simulink model "main_sim"  (R2021a)
settings: Solver=FixedStepAuto  StartTime=0  StopTime=11.0  FixedStep=1e-2  RelTol=1e-3
values from neighbouring files (symbols this model uses):
  Af = 1.6 + 0.00056 * (M-765)    (= 1.7316)    [main.m]    (also in perc_neg_forces.m)
  Cd = 0.27    [main.m]    (also in perc_neg_forces.m)
  Cf = Csigma    (= 40000)    [main.m]    (also in perc_neg_forces.m)
  Cr = Csigma    (= 40000)    [main.m]    (also in perc_neg_forces.m)
  f = 0.015    [main.m]    (also in perc_neg_forces.m)
  g = 9.81    [main.m]    (also in perc_neg_forces.m)
  h = 0.292*2    (= 0.584)    [main.m]    (also in perc_neg_forces.m)
  haero = 0.292*2    (= 0.584)    [main.m]    (also in perc_neg_forces.m)
  Lf = 0.74    [main.m]    (also in perc_neg_forces.m)
  Lr = 0.6    [main.m]    (also in perc_neg_forces.m)
  M = 1000    [main.m]    (also in perc_neg_forces.m)
  reff = ( asin(acos(rstat/rw)) / acos(rstat/rw)) * rw    [main.m]    (also in perc_neg_forces.m)
  rho = 1.225    [main.m]    (also in perc_neg_forces.m)
  Vwind = 5.5    [main.m]    (also in perc_neg_forces.m)
  w_cte = 5    [main.m]    (also in perc_neg_forces.m = w(i))
libraries: simulink x6
settings Model: Creator=joaofonseca  LastModifiedBy=joaofonseca

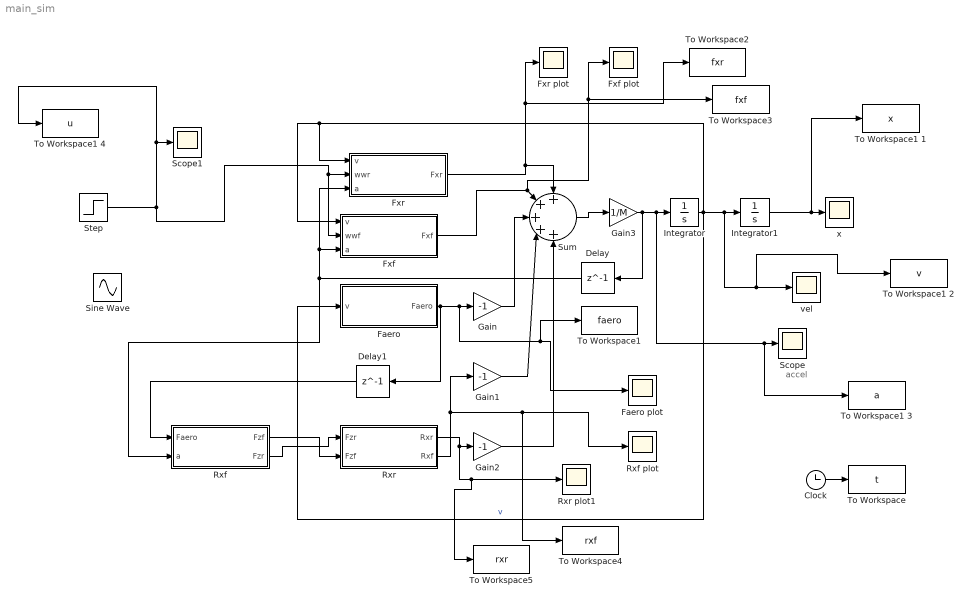
== system main_sim ==
  note: accel
  Clock : Clock
  Delay : Delay  DelayLength=1  InitialCondition=0
  Delay1 : Delay  DelayLength=1  InitialCondition=0
  Faero : Subsystem
  Faero plot : Scope
  Fxf : Subsystem
  Fxf plot : Scope
  Fxr : Subsystem
  Fxr plot : Scope
  Gain : Gain  Gain=-1
  Gain1 : Gain  Gain=-1
  Gain2 : Gain  Gain=-1
  Gain3 : Gain  Gain=1/M
  Integrator : Integrator
  Integrator1 : Integrator  InitialCondition=-2
  Rxf : Subsystem
  Rxf plot : Scope
  Rxr : Subsystem
  Rxr plot1 : Scope
  Scope : Scope
  Scope1 : Scope
  Sine Wave : Sin  Amplitude=25  Bias=26  Frequency=0.5  SampleTime=0
  Step : Step  Time=0  After=w_cte  SampleTime=0
  Sum : Sum  Inputs=+|+|+|+|+
  To Workspace : ToWorkspace  VariableName=t  SampleTime=-1
  To Workspace1 : ToWorkspace  VariableName=faero  SampleTime=-1
  To Workspace1 1 : ToWorkspace  VariableName=x  SampleTime=-1
  To Workspace1 2 : ToWorkspace  VariableName=v  SampleTime=-1
  To Workspace1 3 : ToWorkspace  VariableName=a  SampleTime=-1
  To Workspace1 4 : ToWorkspace  VariableName=u  SampleTime=-1
  To Workspace2 : ToWorkspace  VariableName=fxr  SampleTime=-1
  To Workspace3 : ToWorkspace  VariableName=fxf  SampleTime=-1
  To Workspace4 : ToWorkspace  VariableName=rxf  SampleTime=-1
  To Workspace5 : ToWorkspace  VariableName=rxr  SampleTime=-1
  vel : Scope
  x : Scope
  wires:
  Integrator/1 -> Faero/1(v), To Workspace1 2/1, vel/1, Integrator1/1, Fxf/1(v), Fxr/1(v)  "v"
  Faero/1(Faero) -> Delay1/1, To Workspace1/1, Faero plot/1, Gain/1
  Gain2/1 -> Sum/5
  Gain1/1 -> Sum/4
  Gain/1 -> Sum/3
  Fxf/1(Fxf) -> To Workspace3/1, Fxf plot/1, Sum/2
  Fxr/1(Fxr) -> To Workspace2/1, Fxr plot/1, Sum/1
  Gain3/1 -> Delay/1, To Workspace1 3/1, Scope/1, Integrator/1
  Sum/1 -> Gain3/1
  Rxr/1(Rxr) -> To Workspace5/1, Rxr plot1/1, Gain2/1
  Integrator1/1 -> To Workspace1 1/1, x/1
  Delay/1 -> Rxf/2(a), Fxf/3(a), Fxr/3(a)
  Step/1 -> Fxf/2(wwf), Fxr/2(wwr), To Workspace1 4/1, Scope1/1
  Rxf/1(Fzf) -> Rxr/2(Fzf)
  Rxf/2(Fzr) -> Rxr/1(Fzr)
  Delay1/1 -> Rxf/1(Faero)
  Rxr/2(Rxf) -> To Workspace4/1, Rxf plot/1, Gain1/1
  Clock/1 -> To Workspace/1

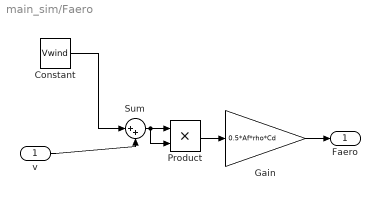
== system main_sim/Faero ==
  v : Inport
  Constant : Constant  Value=Vwind
  Gain : Gain  Gain=0.5*Af*rho*Cd
  Product : Product
  Sum : Sum  Inputs=|++
  Faero : Outport
  wires:
  Constant/1 -> Sum/1
  v/1 -> Sum/2
  Sum/1 -> Product/2, Product/1
  Product/1 -> Gain/1
  Gain/1 -> Faero/1

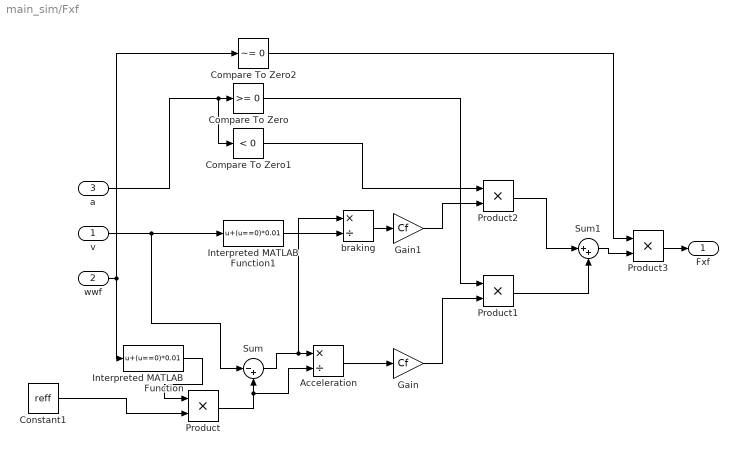
== system main_sim/Fxf ==
  v : Inport
  wwf : Inport  Port=2
  a : Inport  Port=3
  Acceleration : Product  Inputs=*/  OutMax=0.1
  Compare To Zero : simulink/Logic and Bit Operations/Compare To Zero  relop=>=  OutDataTypeStr=uint8  ZeroCross=off
  Compare To Zero1 : simulink/Logic and Bit Operations/Compare To Zero  relop=<  OutDataTypeStr=uint8  ZeroCross=off
  Compare To Zero2 : simulink/Logic and Bit Operations/Compare To Zero  relop=~=  OutDataTypeStr=uint8  ZeroCross=off
  Constant1 : Constant  Value=reff
  Gain : Gain  Gain=Cf
  Gain1 : Gain  Gain=Cf
  Interpreted MATLAB Function : MATLABFcn  MATLABFcn=u+(u==0)*0.01
  Interpreted MATLAB Function1 : MATLABFcn  MATLABFcn=u+(u==0)*0.01
  Product : Product  OutMin=0.0001
  Product1 : Product
  Product2 : Product
  Product3 : Product
  Sum : Sum  Inputs=|-+
  Sum1 : Sum  Inputs=|++
  braking : Product  Inputs=*/
  Fxf : Outport
  wires:
  Product1/1 -> Sum1/2
  Compare To Zero1/1 -> Product2/1
  Constant1/1 -> Product/2
  Product2/1 -> Sum1/1
  Product/1 -> Acceleration/2, Sum/2
  a/1 -> Compare To Zero1/1, Compare To Zero/1
  Sum/1 -> braking/1, Acceleration/1
  Compare To Zero/1 -> Product1/1
  Acceleration/1 -> Gain/1
  Gain1/1 -> Product2/2
  braking/1 -> Gain1/1
  v/1 -> Interpreted MATLAB Function1/1, Sum/1
  Gain/1 -> Product1/2
  Interpreted MATLAB Function/1 -> Product/1
  Interpreted MATLAB Function1/1 -> braking/2
  Compare To Zero2/1 -> Product3/1
  wwf/1 -> Compare To Zero2/1, Interpreted MATLAB Function/1
  Sum1/1 -> Product3/2
  Product3/1 -> Fxf/1

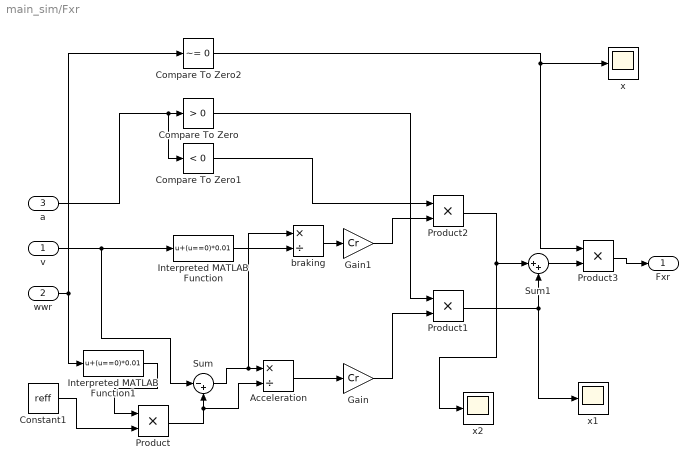
== system main_sim/Fxr ==
  v : Inport
  wwr : Inport  Port=2
  a : Inport  Port=3
  Acceleration : Product  Inputs=*/
  Compare To Zero : simulink/Logic and Bit Operations/Compare To Zero  relop=>  OutDataTypeStr=uint8  ZeroCross=off
  Compare To Zero1 : simulink/Logic and Bit Operations/Compare To Zero  relop=<  OutDataTypeStr=uint8  ZeroCross=off
  Compare To Zero2 : simulink/Logic and Bit Operations/Compare To Zero  relop=~=  OutDataTypeStr=uint8  ZeroCross=off
  Constant1 : Constant  Value=reff
  Gain : Gain  Gain=Cr
  Gain1 : Gain  Gain=Cr
  Interpreted MATLAB Function : MATLABFcn  MATLABFcn=u+(u==0)*0.01
  Interpreted MATLAB Function1 : MATLABFcn  MATLABFcn=u+(u==0)*0.01
  Product{,1..3} (4 alike) : Product
  Sum : Sum  Inputs=|-+
  Sum1 : Sum  Inputs=|++
  braking : Product  Inputs=*/
  x : Scope
  x1 : Scope
  x2 : Scope
  Fxr : Outport
  wires:
  a/1 -> Compare To Zero1/1, Compare To Zero/1
  Constant1/1 -> Product/2
  Product/1 -> Acceleration/2, Sum/2
  v/1 -> Interpreted MATLAB Function/1, Sum/1
  Sum/1 -> braking/1, Acceleration/1
  Acceleration/1 -> Gain/1
  Gain/1 -> Product1/2
  Compare To Zero/1 -> Product1/1
  Product1/1 -> x1/1, Sum1/2
  braking/1 -> Gain1/1
  Compare To Zero1/1 -> Product2/1
  Gain1/1 -> Product2/2
  Product2/1 -> x2/1, Sum1/1
  Interpreted MATLAB Function/1 -> braking/2
  wwr/1 -> Compare To Zero2/1, Interpreted MATLAB Function1/1
  Interpreted MATLAB Function1/1 -> Product/1
  Sum1/1 -> Product3/2
  Compare To Zero2/1 -> Product3/1, x/1
  Product3/1 -> Fxr/1

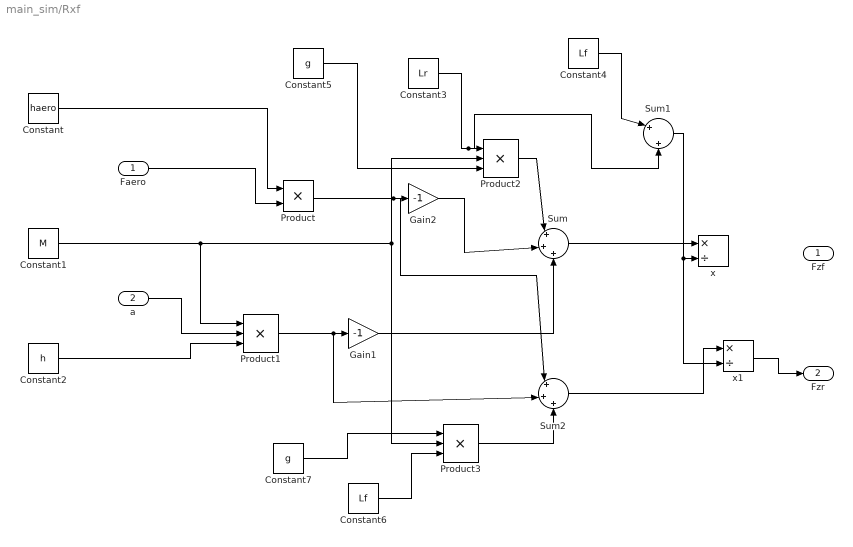
== system main_sim/Rxf ==
  Faero : Inport
  a : Inport  Port=2
  Constant : Constant  Value=haero
  Constant1 : Constant  Value=M
  Constant2 : Constant  Value=h
  Constant3 : Constant  Value=Lr
  Constant4 : Constant  Value=Lf
  Constant5 : Constant  Value=g
  Constant6 : Constant  Value=Lf
  Constant7 : Constant  Value=g
  Gain1 : Gain  Gain=-1
  Gain2 : Gain  Gain=-1
  Product : Product
  Product1 : Product  Inputs=3
  Product2 : Product  Inputs=3
  Product3 : Product  Inputs=3
  Sum : Sum  Inputs=|+|+|+
  Sum1 : Sum  Inputs=|+|+
  Sum2 : Sum  Inputs=|+|+|+
  x : Product  Inputs=*/
  x1 : Product  Inputs=*/
  Fzf : Outport
  Fzr : Outport  Port=2
  wires:
  Faero/1 -> Product/2
  Constant/1 -> Product/1
  Constant1/1 -> Product3/2, Product2/2, Product1/1
  a/1 -> Product1/2
  Constant2/1 -> Product1/3
  Product1/1 -> Sum2/2, Gain1/1
  Constant3/1 -> Sum1/2, Product2/1
  Constant5/1 -> Product2/3
  Product2/1 -> Sum/1
  Product/1 -> Sum2/1, Gain2/1
  Gain1/1 -> Sum/3
  Sum/1 -> x/1
  Constant4/1 -> Sum1/1
  Sum1/1 -> x1/2, x/2
  Gain2/1 -> Sum/2
  Constant6/1 -> Product3/3
  Constant7/1 -> Product3/1
  Product3/1 -> Sum2/3
  Sum2/1 -> x1/1
  x1/1 -> Fzr/1

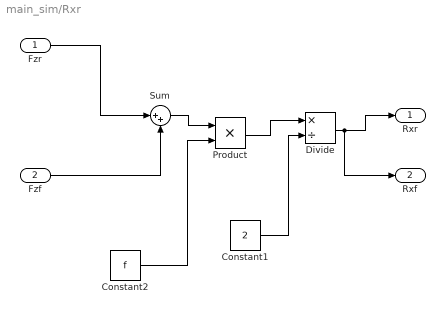
== system main_sim/Rxr ==
  Fzr : Inport
  Fzf : Inport  Port=2
  Constant1 : Constant  Value=2
  Constant2 : Constant  Value=f
  Divide : Product  Inputs=*/
  Product : Product
  Sum : Sum  Inputs=|++
  Rxr : Outport
  Rxf : Outport  Port=2
  wires:
  Fzf/1 -> Sum/2
  Fzr/1 -> Sum/1
  Sum/1 -> Product/1
  Constant2/1 -> Product/2
  Product/1 -> Divide/1
  Constant1/1 -> Divide/2
  Divide/1 -> Rxf/1, Rxr/1
